simulink model "PID_IMC"  (R2022a)
settings: Solver=VariableStepAuto  StartTime=0.0  StopTime=30  RelTol=1e-3
libraries: cstblocks x4
settings Model: Creator=dsolorzano  LastModifiedBy=carlo

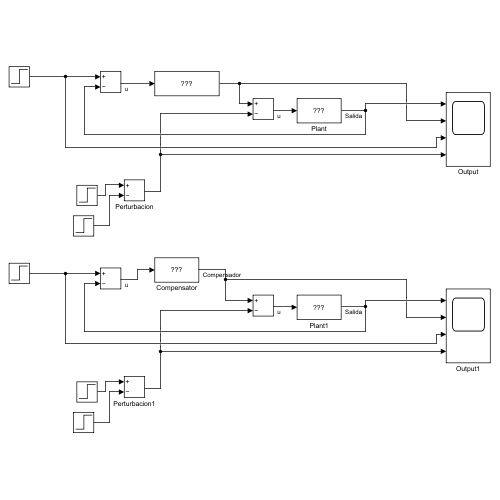
[thumbnail: Simulink's stored preview of the top-level diagram]
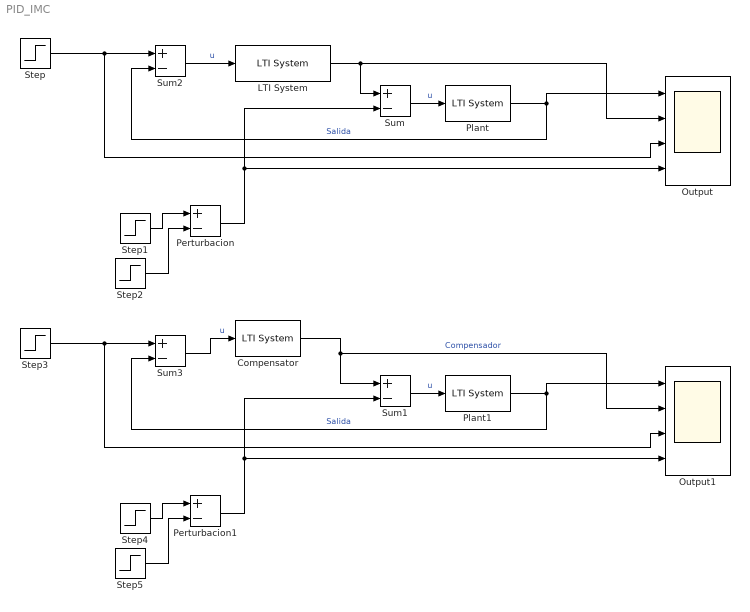
== system PID_IMC ==
  Compensator : cstblocks/LTI System  sys=C  IC=[]
  LTI System : cstblocks/LTI System  sys=pid1  IC=[]
  Output : Scope  NumInputPorts=4
  Output1 : Scope  NumInputPorts=4
  Perturbacion : Sum  Inputs=+-
  Perturbacion1 : Sum  Inputs=+-
  Plant : cstblocks/LTI System  sys=G  IC=[]
  Plant1 : cstblocks/LTI System  sys=G  IC=[]
  Step : Step  After=0.6  SampleTime=0
  Step1 : Step  Time=8  After=0.05  SampleTime=0
  Step2 : Step  Time=15  After=0.05  SampleTime=0
  Step3 : Step  After=0.6  SampleTime=0
  Step4 : Step  Time=8  After=0.05  SampleTime=0
  Step5 : Step  Time=15  After=0.05  SampleTime=0
  Sum{,1..3} (4 alike) : Sum  Inputs=+-
  wires:
  Plant/1 -> Sum2/2, Output/1  "Salida"
  Step1/1 -> Perturbacion/1
  Step2/1 -> Perturbacion/2
  Perturbacion/1 -> Sum/2, Output/4
  Step/1 -> Sum2/1, Output/3
  Sum/1 -> Plant/1  "u"
  Sum2/1 -> LTI System/1  "u"
  LTI System/1 -> Output/2, Sum/1
  Sum1/1 -> Plant1/1  "u"
  Step4/1 -> Perturbacion1/1
  Step3/1 -> Sum3/1, Output1/3
  Step5/1 -> Perturbacion1/2
  Perturbacion1/1 -> Sum1/2, Output1/4
  Plant1/1 -> Sum3/2, Output1/1  "Salida"
  Sum3/1 -> Compensator/1  "u"
  Compensator/1 -> Output1/2, Sum1/1  "Compensador"
